simulink model "rSOC"  (R2024b)
settings: configuration reference "STM32H7_Config" (kept outside this file)
undefined symbols (not defined in the file): EAccumulatorCapacity, QAccumulatorCapacity, tSystemsTask
settings Model: DataDictionary=Master_Dictionary.sldd  EnableAccessToBaseWorkspace=off  Creator=torni  LastModifiedBy=William
settings ConfigSetRef: SourceName=STM32H7_Config

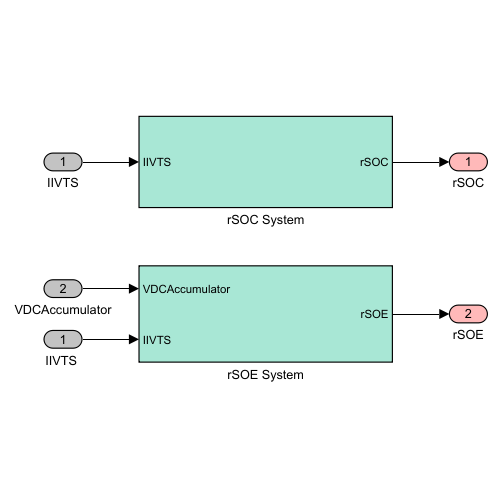
[thumbnail: Simulink's stored preview of the top-level diagram]
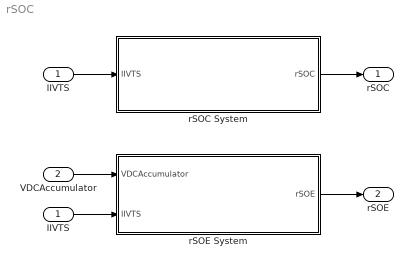
== system rSOC ==
  IIVTS : Inport  OutDataTypeStr=double
  VDCAccumulator : Inport  Port=2  OutDataTypeStr=double
  "IIVTS " : InportShadow  OutDataTypeStr=double
  rSOC System : Subsystem
  rSOE System : Subsystem
  rSOC : Outport  OutDataTypeStr=double  VectorParamsAs1DForOutWhenUnconnected=off
  rSOE : Outport  Port=2  OutDataTypeStr=double  VectorParamsAs1DForOutWhenUnconnected=off
  wires:
  IIVTS/1 -> rSOC System/1(IIVTS)
  rSOC System/1(rSOC) -> rSOC/1
  rSOE System/1(rSOE) -> rSOE/1
  VDCAccumulator/1 -> rSOE System/1(VDCAccumulator)
  "IIVTS "/1 -> rSOE System/2(IIVTS)

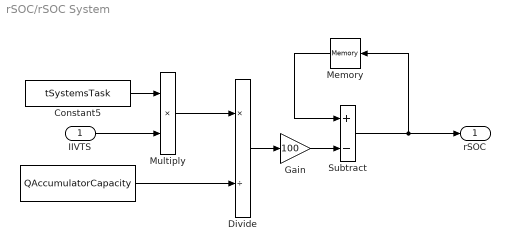
== system rSOC/rSOC System ==
  IIVTS : Inport  OutDataTypeStr=double
  " " : Constant  Value=QAccumulatorCapacity
  Constant5 : Constant  Value=tSystemsTask
  Divide : Product  Inputs=*/
  Gain : Gain  Gain=100
  Memory : Memory  InitialCondition=100  InheritSampleTime=on
  Multiply : Product
  Subtract : Sum  Inputs=+-
  rSOC : Outport  OutDataTypeStr=double  VectorParamsAs1DForOutWhenUnconnected=off
  wires:
  Memory/1 -> Subtract/1
  Constant5/1 -> Multiply/1
  IIVTS/1 -> Multiply/2
  Multiply/1 -> Divide/1
  Subtract/1 -> rSOC/1, Memory/1
  Divide/1 -> Gain/1
  " "/1 -> Divide/2
  Gain/1 -> Subtract/2

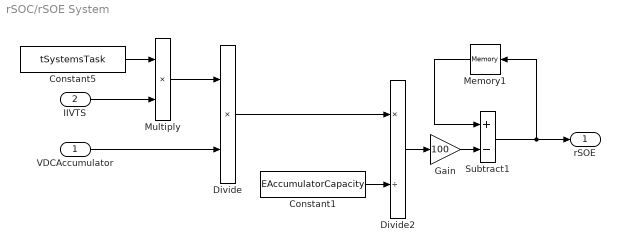
== system rSOC/rSOE System ==
  VDCAccumulator : Inport  OutDataTypeStr=double
  IIVTS : Inport  Port=2  OutDataTypeStr=double
  Constant1 : Constant  Value=EAccumulatorCapacity
  Constant5 : Constant  Value=tSystemsTask
  Divide : Product  Inputs=**
  Divide2 : Product  Inputs=*/
  Gain : Gain  Gain=100
  Memory1 : Memory  InitialCondition=100  InheritSampleTime=on
  Multiply : Product
  Subtract1 : Sum  Inputs=+-
  rSOE : Outport  OutDataTypeStr=double  VectorParamsAs1DForOutWhenUnconnected=off
  wires:
  VDCAccumulator/1 -> Divide/2
  Divide/1 -> Divide2/1
  Divide2/1 -> Gain/1
  Memory1/1 -> Subtract1/1
  Subtract1/1 -> rSOE/1, Memory1/1
  Constant5/1 -> Multiply/1
  Multiply/1 -> Divide/1
  IIVTS/1 -> Multiply/2
  Constant1/1 -> Divide2/2
  Gain/1 -> Subtract1/2
